simulink model "test"  (R2024b)
settings: Solver=VariableStepAuto  StartTime=0.0  StopTime=10.0  RelTol=1e-3
libraries: fl_lib x5
settings Model: Creator=leo  LastModifiedBy=leo

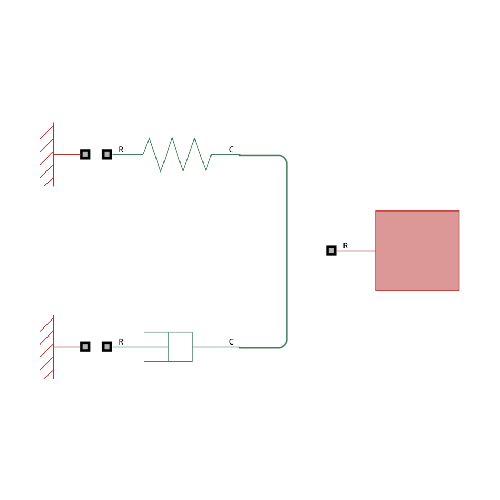
[thumbnail: Simulink's stored preview of the top-level diagram]
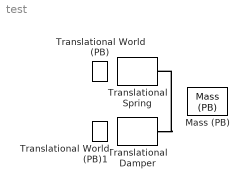
== system test ==
  Mass (PB) : fl_lib/Translational/Elements/Mass (PB)  mass=1 kg  v_specify=off  v_priority=High  v=0 m/s  v_nominal_specify=off  v_nominal_value=1  v_nominal_unit=m/s  f_acc_specify=off  f_acc_priority=None  f_acc=0 N  f_acc_nominal_specify=off  f_acc_nominal_value=1  f_acc_nominal_unit=N  f_specify=off  f_priority=None  f=0 N  f_nominal_specify=off  f_nominal_value=1  f_nominal_unit=N
      settings: InternalSimscapePortConfiguration="{\"Bottom\":[],\"Left\":[{\"id\":\"R\",\"label\":\"R\",\"type\":\"foundation.translational.translational\"}],\"Right\":[],\"Top\":[]}"
  Translational Damper : fl_lib/Mechanical/Translational Elements/Translational Damper  D=100 N*s/m  v_specify=off  v_priority=None  v=0 m/s  v_nominal_specify=off  v_nominal_value=1  v_nominal_unit=m/s  f_specify=off  f_priority=None  f=0 N  f_nominal_specify=off  f_nominal_value=1  f_nominal_unit=N
  Translational Spring : fl_lib/Mechanical/Translational Elements/Translational Spring  spr_rate=1000 N/m  v_specify=off  v_priority=None  v=0 m/s  v_nominal_specify=off  v_nominal_value=1  v_nominal_unit=m/s  f_specify=off  f_priority=None  f=0 N  f_nominal_specify=off  f_nominal_value=1  f_nominal_unit=N  x_specify=off  x_priority=High  x=0 m  x_nominal_specify=off  x_nominal_value=1  x_nominal_unit=m
  Translational World (PB) : fl_lib/Translational/Elements/Translational World (PB)
      settings: InternalSimscapePortConfiguration="{\"Bottom\":[],\"Left\":[],\"Right\":[{\"id\":\"R\",\"label\":\"\",\"type\":\"foundation.translational.translational\"}],\"Top\":[]}"
  Translational World (PB)1 : fl_lib/Translational/Elements/Translational World (PB)
      settings: InternalSimscapePortConfiguration="{\"Bottom\":[],\"Left\":[],\"Right\":[{\"id\":\"R\",\"label\":\"\",\"type\":\"foundation.translational.translational\"}],\"Top\":[]}"
  connections:
  Translational Damper/RConn1 -- Translational Spring/RConn1
